simulink model "Final_world"  (R2020a)
settings: Solver=VariableStepAuto  StartTime=0.0  StopTime=10.0  RelTol=1e-3
libraries: vrlib x6
settings Model: Creator=Praneet Nayak  LastModifiedBy=Praneet Nayak

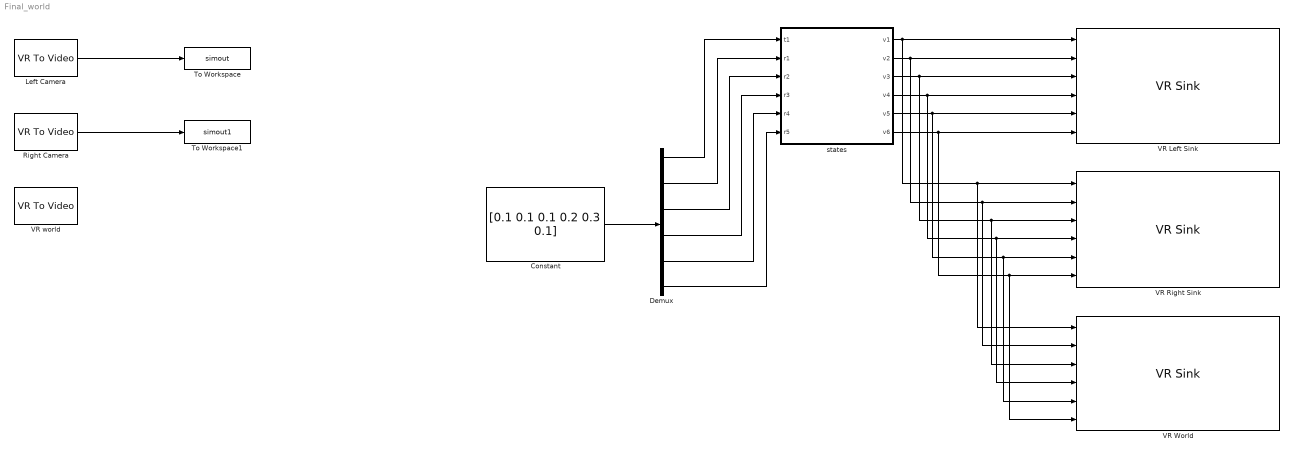
== system Final_world ==
  Constant : Constant  Value=[0.1 0.1 0.1 0.2 0.3 0.1]
  Demux : Demux  Outputs=6
  Left Camera : vrlib/VR To Video  InstantiateOnLoad=on  SampleTime=0.1  ViewEnable=on  RemoteChange=off  RemoteView=off  WorldFileName=jlr_world_final2_left.x3d  WorldDescription=Straight Road Strip - 2 Lanes  AutoView=off  VideoDimensions=[1080 1920]  AllowVariableSize=off
      settings: SourceProductBaseCode=SL
  Right Camera : vrlib/VR To Video  InstantiateOnLoad=on  SampleTime=0.1  ViewEnable=on  RemoteChange=off  RemoteView=off  WorldFileName=jlr_world_final2_right.x3d  WorldDescription=Straight Road Strip - 2 Lanes  AutoView=off  VideoDimensions=[1080 1920]  AllowVariableSize=off
      settings: SourceProductBaseCode=SL
  To Workspace : ToWorkspace  VariableName=simout  SaveFormat=Timeseries  SampleTime=-1
  To Workspace1 : ToWorkspace  VariableName=simout1  SaveFormat=Timeseries  SampleTime=-1
  VR Left Sink : vrlib/VR Sink  InstantiateOnLoad=on  SampleTime=0.1  ViewEnable=on  RemoteChange=off  RemoteView=off  FieldsWritten=axis_Trans1.translation.3.1.1.double#axis_Rev1.rotation.4.1.1.double#axis_Rev2.rotation.4.1.1.double#axis_Rev3.rotation.4.1.1.double#axis_Rev4.rotation.4.1.1.double#axis_Rev5.rotation.4.1.1.double  WorldFileName=jlr_world_final2_left.x3d  WorldDescription=Straight Road Strip - 2 Lanes  AutoView=off  VideoDimensions=[]  AllowVariableSize=off
  VR Right Sink : vrlib/VR Sink  InstantiateOnLoad=on  SampleTime=0.1  ViewEnable=on  RemoteChange=off  RemoteView=off  FieldsWritten=axis_Trans1.translation.3.1.1.double#axis_Rev1.rotation.4.1.1.double#axis_Rev2.rotation.4.1.1.double#axis_Rev3.rotation.4.1.1.double#axis_Rev4.rotation.4.1.1.double#axis_Rev5.rotation.4.1.1.double  WorldFileName=jlr_world_final2_right.x3d  WorldDescription=Straight Road Strip - 2 Lanes  AutoView=off  VideoDimensions=[]  AllowVariableSize=off
  VR World : vrlib/VR Sink  InstantiateOnLoad=on  SampleTime=0.1  ViewEnable=on  RemoteChange=off  RemoteView=off  FieldsWritten=axis_Trans1.translation.3.1.1.double#axis_Rev1.rotation.4.1.1.double#axis_Rev2.rotation.4.1.1.double#axis_Rev3.rotation.4.1.1.double#axis_Rev4.rotation.4.1.1.double#axis_Rev5.rotation.4.1.1.double  WorldFileName=jlr_world_final2.x3d  WorldDescription=Straight Road Strip - 2 Lanes  AutoView=off  VideoDimensions=[]  AllowVariableSize=off
  VR world : vrlib/VR To Video  InstantiateOnLoad=on  SampleTime=0.1  ViewEnable=on  RemoteChange=off  RemoteView=off  WorldFileName=jlr_world_final2.x3d  WorldDescription=Straight Road Strip - 2 Lanes  AutoView=off  VideoDimensions=[1080 1920]  AllowVariableSize=off
      settings: SourceProductBaseCode=SL
  states : MATLAB Function  TreatAsAtomicUnit=on
  wires:
  Left Camera/1 -> To Workspace/1
  Right Camera/1 -> To Workspace1/1
  Constant/1 -> Demux/1
  Demux/1 -> states/1(t1)
  Demux/2 -> states/2(r1)
  Demux/3 -> states/3(r2)
  Demux/4 -> states/4(r3)
  Demux/5 -> states/5(r4)
  Demux/6 -> states/6(r5)
  states/1(v1) -> VR Left Sink/1, VR Right Sink/1, VR World/1
  states/2(v2) -> VR Left Sink/2, VR World/2, VR Right Sink/2
  states/3(v3) -> VR Left Sink/3, VR World/3, VR Right Sink/3
  states/4(v4) -> VR Left Sink/4, VR World/4, VR Right Sink/4
  states/5(v5) -> VR Left Sink/5, VR World/5, VR Right Sink/5
  states/6(v6) -> VR Left Sink/6, VR World/6, VR Right Sink/6

== matlab function Final_world/states ==
  data: t1 input; v1 output; r1 input; r2 input; r3 input; r4 input; r5 input; v2 output; v3 output; v4 output; v5 output; v6 output
function [v1,v2,v3,v4,v5,v6] = fcn(t1,r1,r2,r3,r4,r5)
v1 = [0 -t1 0];
v2 = [0 0 -1 r1];
v3 = [0 0 -1 r2];
v4 = [1 0 0 r3];
v5 = [0.16232 0.077123 0.98372 -r4];
v6 = [1 0 0 r5];
